simulink model "FSK"  (R2018b)
settings: Solver=FixedStepAuto  StartTime=0.0  StopTime=10.0  FixedStep=0.01  RelTol=1e-3
settings Model: Creator=root  LastModifiedBy=root

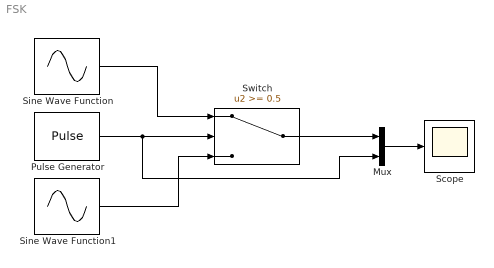
== system FSK ==
  Mux : Mux  Inputs=2
  Pulse Generator : DiscretePulseGenerator  PulseType=Time based  PulseWidth=50
  Scope : Scope
  Sine Wave Function : Sin  Frequency=2*pi*4  SampleTime=0.01
  Sine Wave Function1 : Sin  Frequency=2*pi*2  SampleTime=0.01
  Switch : Switch  Threshold=0.5
  wires:
  Switch/1 -> Mux/1
  Pulse Generator/1 -> Mux/2, Switch/2
  Sine Wave Function/1 -> Switch/1
  Sine Wave Function1/1 -> Switch/3
  Mux/1 -> Scope/1
